simulink model "Channelizer_rb_v1"  (R2023b)
settings: Solver=VariableStepAuto  StartTime=0.0  StopTime=2048  RelTol=1e-3
PostLoadFcn:
  | TT = numerictype(1,16,15);
  | FF = fimath('RoundingMethod','Nearest','OverflowAction','Saturate');
  | mdl = channelizer_init(TT, FF);
  | channelizer = channelizer_model(mdl, TT, FF );
  | ch15 = 1; ch14 = ch15; ch13 = ch14; ch12 = ch13;
  | ch11 = ch12; ch10 = ch11; ch9 = ch10; ch8 = ch9;
  | ch7 = ch8; ch6 = ch7; ch5 = ch6; ch4 = ch5;
  | ch3 = ch4; ch2 = ch3; ch1 = ch2; ch0 = ch1;
undefined symbols (not defined in the file or in its folder): S, vsva2197, xcvc1902
libraries: aieUtilities x39, aieBasic x34, commrflib2 x16, commfilt2 x16, hlsBasic x3, vmcUtilities x1, commchan3 x1, commrandsrc3 x1, commdigbbndam3 x1
(part 2 of 2)

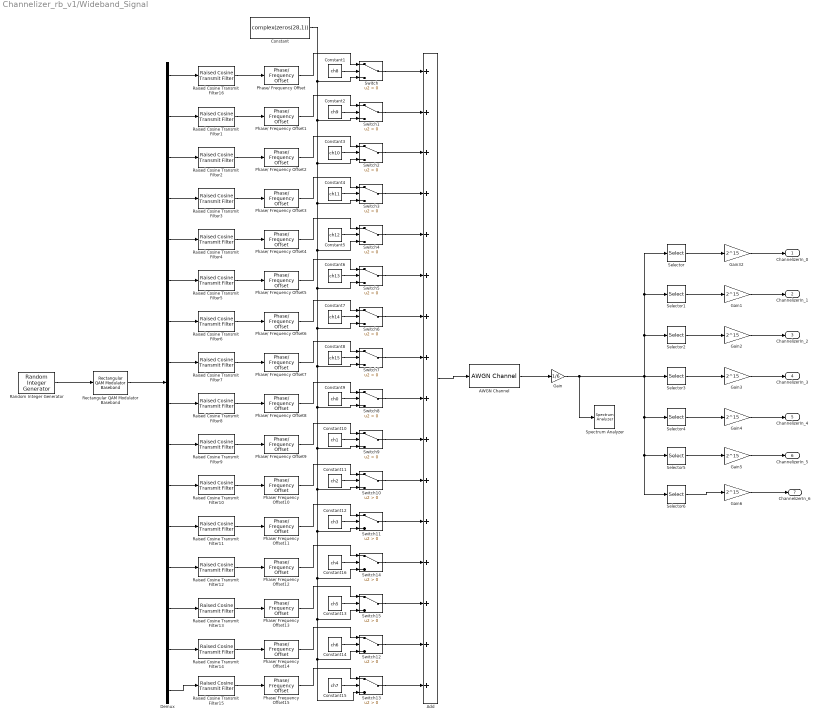
== system Channelizer_rb_v1/Wideband_Signal ==
  AWGN Channel : commchan3/AWGN Channel  LegacyMode=off  NoiseMethod="Signal to noise ratio  (SNR)"  noiseMode="Signal to noise ratio  (SNR)"  EbNo=10  EsNo=10  SNR=20  BitsPerSymbol=1  SignalPower=1  SamplesPerSymbol=1  SymbolPeriod=1  VarianceSource=Parameter  Variance=1  RandomStream=Global stream  Seed=67  SimulateUsing=Code generation
  Add : Sum  Inputs=++++++++++++++++
  Constant : Constant  Value=complex(zeros(28,1))
  Constant1 : Constant  Value=ch8
  Constant10 : Constant  Value=ch1
  Constant11 : Constant  Value=ch2
  Constant12 : Constant  Value=ch3
  Constant13 : Constant  Value=ch5
  Constant14 : Constant  Value=ch6
  Constant15 : Constant  Value=ch7
  Constant16 : Constant  Value=ch4
  Constant2 : Constant  Value=ch9
  Constant3 : Constant  Value=ch10
  Constant4 : Constant  Value=ch11
  Constant5 : Constant  Value=ch12
  Constant6 : Constant  Value=ch13
  Constant7 : Constant  Value=ch14
  Constant8 : Constant  Value=ch15
  Constant9 : Constant  Value=ch0
  Demux : Demux  Outputs=16
  Gain : Gain  Gain=1/6
  Gain{1..6,32} (7 alike) : Gain  Gain=2^15  OutDataTypeStr=int16
  Phase/ Frequency Offset : commrflib2/Phase// Frequency Offset  phaseOffset=0  freqPort=off  freqOffset=-8 * 8.75e9 / 16
  Phase/ Frequency Offset1 : commrflib2/Phase// Frequency Offset  phaseOffset=0  freqPort=off  freqOffset=-7 * 8.75e9 / 16
  Phase/ Frequency Offset10 : commrflib2/Phase// Frequency Offset  phaseOffset=0  freqPort=off  freqOffset=2 * 8.75e9 / 16
  Phase/ Frequency Offset11 : commrflib2/Phase// Frequency Offset  phaseOffset=0  freqPort=off  freqOffset=3 * 8.75e9 / 16
  Phase/ Frequency Offset12 : commrflib2/Phase// Frequency Offset  phaseOffset=0  freqPort=off  freqOffset=4 * 8.75e9 / 16
  Phase/ Frequency Offset13 : commrflib2/Phase// Frequency Offset  phaseOffset=0  freqPort=off  freqOffset=5 * 8.75e9 / 16
  Phase/ Frequency Offset14 : commrflib2/Phase// Frequency Offset  phaseOffset=0  freqPort=off  freqOffset=6 * 8.75e9 / 16
  Phase/ Frequency Offset15 : commrflib2/Phase// Frequency Offset  phaseOffset=0  freqPort=off  freqOffset=7 * 8.75e9 / 16
  Phase/ Frequency Offset2 : commrflib2/Phase// Frequency Offset  phaseOffset=0  freqPort=off  freqOffset=-6 * 8.75e9 / 16
  Phase/ Frequency Offset3 : commrflib2/Phase// Frequency Offset  phaseOffset=0  freqPort=off  freqOffset=-5 * 8.75e9 / 16
  Phase/ Frequency Offset4 : commrflib2/Phase// Frequency Offset  phaseOffset=0  freqPort=off  freqOffset=-4 * 8.75e9 / 16
  Phase/ Frequency Offset5 : commrflib2/Phase// Frequency Offset  phaseOffset=0  freqPort=off  freqOffset=-3 * 8.75e9 / 16
  Phase/ Frequency Offset6 : commrflib2/Phase// Frequency Offset  phaseOffset=0  freqPort=off  freqOffset=-2 * 8.75e9 / 16
  Phase/ Frequency Offset7 : commrflib2/Phase// Frequency Offset  phaseOffset=0  freqPort=off  freqOffset=-1 * 8.75e9 / 16
  Phase/ Frequency Offset8 : commrflib2/Phase// Frequency Offset  phaseOffset=0  freqPort=off  freqOffset=0 * 8.75e9 / 16
  Phase/ Frequency Offset9 : commrflib2/Phase// Frequency Offset  phaseOffset=0  freqPort=off  freqOffset=1 * 8.75e9 / 16
  Raised Cosine Transmit Filter1 : commfilt2/Raised Cosine Transmit Filter  filtType=Normal  R=0.3  filtSpan=10  N=28  filterGain=1  InputProcessing=Columns as channels (frame based)  RateOptions=Enforce single-rate processing  framing=Mute  checkCoeff=off  variableName=rcTxFilt1  checkGain=Normalized  sampMode=Mute  saveAsFlag=0  currentFiltSpan=10  D=(10)/2  launchFVT=on  roundingMode=Floor  overflowMode=off  coeffDataTypeStr=Inherit: Same word length as input  coeffMin=[]  coeffMax=[]  coeffLastDataTypeStr=Inherit: Same word length as input  outputDataTypeStr=Inherit: Same as accumulator  outputMin=[]  outputMax=[]  outputLastDataTypeStr=Inherit: Same as accumulator
  Raised Cosine Transmit Filter10 : commfilt2/Raised Cosine Transmit Filter  filtType=Normal  R=0.3  filtSpan=10  N=28  filterGain=1  InputProcessing=Columns as channels (frame based)  RateOptions=Enforce single-rate processing  framing=Mute  checkCoeff=off  variableName=rcTxFilt10  checkGain=Normalized  sampMode=Mute  saveAsFlag=0  currentFiltSpan=10  D=(10)/2  launchFVT=on  roundingMode=Floor  overflowMode=off  coeffDataTypeStr=Inherit: Same word length as input  coeffMin=[]  coeffMax=[]  coeffLastDataTypeStr=Inherit: Same word length as input  outputDataTypeStr=Inherit: Same as accumulator  outputMin=[]  outputMax=[]  outputLastDataTypeStr=Inherit: Same as accumulator
  Raised Cosine Transmit Filter11 : commfilt2/Raised Cosine Transmit Filter  filtType=Normal  R=0.3  filtSpan=10  N=28  filterGain=1  InputProcessing=Columns as channels (frame based)  RateOptions=Enforce single-rate processing  framing=Mute  checkCoeff=off  variableName=rcTxFilt11  checkGain=Normalized  sampMode=Mute  saveAsFlag=0  currentFiltSpan=10  D=(10)/2  launchFVT=on  roundingMode=Floor  overflowMode=off  coeffDataTypeStr=Inherit: Same word length as input  coeffMin=[]  coeffMax=[]  coeffLastDataTypeStr=Inherit: Same word length as input  outputDataTypeStr=Inherit: Same as accumulator  outputMin=[]  outputMax=[]  outputLastDataTypeStr=Inherit: Same as accumulator
  Raised Cosine Transmit Filter12 : commfilt2/Raised Cosine Transmit Filter  filtType=Normal  R=0.3  filtSpan=10  N=28  filterGain=1  InputProcessing=Columns as channels (frame based)  RateOptions=Enforce single-rate processing  framing=Mute  checkCoeff=off  variableName=rcTxFilt12  checkGain=Normalized  sampMode=Mute  saveAsFlag=0  currentFiltSpan=10  D=(10)/2  launchFVT=on  roundingMode=Floor  overflowMode=off  coeffDataTypeStr=Inherit: Same word length as input  coeffMin=[]  coeffMax=[]  coeffLastDataTypeStr=Inherit: Same word length as input  outputDataTypeStr=Inherit: Same as accumulator  outputMin=[]  outputMax=[]  outputLastDataTypeStr=Inherit: Same as accumulator
  Raised Cosine Transmit Filter13 : commfilt2/Raised Cosine Transmit Filter  filtType=Normal  R=0.3  filtSpan=10  N=28  filterGain=1  InputProcessing=Columns as channels (frame based)  RateOptions=Enforce single-rate processing  framing=Mute  checkCoeff=off  variableName=rcTxFilt13  checkGain=Normalized  sampMode=Mute  saveAsFlag=0  currentFiltSpan=10  D=(10)/2  launchFVT=on  roundingMode=Floor  overflowMode=off  coeffDataTypeStr=Inherit: Same word length as input  coeffMin=[]  coeffMax=[]  coeffLastDataTypeStr=Inherit: Same word length as input  outputDataTypeStr=Inherit: Same as accumulator  outputMin=[]  outputMax=[]  outputLastDataTypeStr=Inherit: Same as accumulator
  Raised Cosine Transmit Filter14 : commfilt2/Raised Cosine Transmit Filter  filtType=Normal  R=0.3  filtSpan=10  N=28  filterGain=1  InputProcessing=Columns as channels (frame based)  RateOptions=Enforce single-rate processing  framing=Mute  checkCoeff=off  variableName=rcTxFilt14  checkGain=Normalized  sampMode=Mute  saveAsFlag=0  currentFiltSpan=10  D=(10)/2  launchFVT=on  roundingMode=Floor  overflowMode=off  coeffDataTypeStr=Inherit: Same word length as input  coeffMin=[]  coeffMax=[]  coeffLastDataTypeStr=Inherit: Same word length as input  outputDataTypeStr=Inherit: Same as accumulator  outputMin=[]  outputMax=[]  outputLastDataTypeStr=Inherit: Same as accumulator
  Raised Cosine Transmit Filter15 : commfilt2/Raised Cosine Transmit Filter  filtType=Normal  R=0.3  filtSpan=10  N=28  filterGain=1  InputProcessing=Columns as channels (frame based)  RateOptions=Enforce single-rate processing  framing=Mute  checkCoeff=off  variableName=rcTxFilt15  checkGain=Normalized  sampMode=Mute  saveAsFlag=0  currentFiltSpan=10  D=(10)/2  launchFVT=on  roundingMode=Floor  overflowMode=off  coeffDataTypeStr=Inherit: Same word length as input  coeffMin=[]  coeffMax=[]  coeffLastDataTypeStr=Inherit: Same word length as input  outputDataTypeStr=Inherit: Same as accumulator  outputMin=[]  outputMax=[]  outputLastDataTypeStr=Inherit: Same as accumulator
  Raised Cosine Transmit Filter16 : commfilt2/Raised Cosine Transmit Filter  filtType=Normal  R=0.3  filtSpan=10  N=28  filterGain=1  InputProcessing=Columns as channels (frame based)  RateOptions=Enforce single-rate processing  framing=Mute  checkCoeff=off  variableName=rcTxFilt16  checkGain=Normalized  sampMode=Mute  saveAsFlag=0  currentFiltSpan=10  D=(10)/2  launchFVT=on  roundingMode=Floor  overflowMode=off  coeffDataTypeStr=Inherit: Same word length as input  coeffMin=[]  coeffMax=[]  coeffLastDataTypeStr=Inherit: Same word length as input  outputDataTypeStr=Inherit: Same as accumulator  outputMin=[]  outputMax=[]  outputLastDataTypeStr=Inherit: Same as accumulator
  Raised Cosine Transmit Filter2 : commfilt2/Raised Cosine Transmit Filter  filtType=Normal  R=0.3  filtSpan=10  N=28  filterGain=1  InputProcessing=Columns as channels (frame based)  RateOptions=Enforce single-rate processing  framing=Mute  checkCoeff=off  variableName=rcTxFilt2  checkGain=Normalized  sampMode=Mute  saveAsFlag=0  currentFiltSpan=10  D=(10)/2  launchFVT=on  roundingMode=Floor  overflowMode=off  coeffDataTypeStr=Inherit: Same word length as input  coeffMin=[]  coeffMax=[]  coeffLastDataTypeStr=Inherit: Same word length as input  outputDataTypeStr=Inherit: Same as accumulator  outputMin=[]  outputMax=[]  outputLastDataTypeStr=Inherit: Same as accumulator
  Raised Cosine Transmit Filter3 : commfilt2/Raised Cosine Transmit Filter  filtType=Normal  R=0.3  filtSpan=10  N=28  filterGain=1  InputProcessing=Columns as channels (frame based)  RateOptions=Enforce single-rate processing  framing=Mute  checkCoeff=off  variableName=rcTxFilt3  checkGain=Normalized  sampMode=Mute  saveAsFlag=0  currentFiltSpan=10  D=(10)/2  launchFVT=on  roundingMode=Floor  overflowMode=off  coeffDataTypeStr=Inherit: Same word length as input  coeffMin=[]  coeffMax=[]  coeffLastDataTypeStr=Inherit: Same word length as input  outputDataTypeStr=Inherit: Same as accumulator  outputMin=[]  outputMax=[]  outputLastDataTypeStr=Inherit: Same as accumulator
  Raised Cosine Transmit Filter4 : commfilt2/Raised Cosine Transmit Filter  filtType=Normal  R=0.3  filtSpan=10  N=28  filterGain=1  InputProcessing=Columns as channels (frame based)  RateOptions=Enforce single-rate processing  framing=Mute  checkCoeff=off  variableName=rcTxFilt4  checkGain=Normalized  sampMode=Mute  saveAsFlag=0  currentFiltSpan=10  D=(10)/2  launchFVT=on  roundingMode=Floor  overflowMode=off  coeffDataTypeStr=Inherit: Same word length as input  coeffMin=[]  coeffMax=[]  coeffLastDataTypeStr=Inherit: Same word length as input  outputDataTypeStr=Inherit: Same as accumulator  outputMin=[]  outputMax=[]  outputLastDataTypeStr=Inherit: Same as accumulator
  Raised Cosine Transmit Filter5 : commfilt2/Raised Cosine Transmit Filter  filtType=Normal  R=0.3  filtSpan=10  N=28  filterGain=1  InputProcessing=Columns as channels (frame based)  RateOptions=Enforce single-rate processing  framing=Mute  checkCoeff=off  variableName=rcTxFilt5  checkGain=Normalized  sampMode=Mute  saveAsFlag=0  currentFiltSpan=10  D=(10)/2  launchFVT=on  roundingMode=Floor  overflowMode=off  coeffDataTypeStr=Inherit: Same word length as input  coeffMin=[]  coeffMax=[]  coeffLastDataTypeStr=Inherit: Same word length as input  outputDataTypeStr=Inherit: Same as accumulator  outputMin=[]  outputMax=[]  outputLastDataTypeStr=Inherit: Same as accumulator
  Raised Cosine Transmit Filter6 : commfilt2/Raised Cosine Transmit Filter  filtType=Normal  R=0.3  filtSpan=10  N=28  filterGain=1  InputProcessing=Columns as channels (frame based)  RateOptions=Enforce single-rate processing  framing=Mute  checkCoeff=off  variableName=rcTxFilt6  checkGain=Normalized  sampMode=Mute  saveAsFlag=0  currentFiltSpan=10  D=(10)/2  launchFVT=on  roundingMode=Floor  overflowMode=off  coeffDataTypeStr=Inherit: Same word length as input  coeffMin=[]  coeffMax=[]  coeffLastDataTypeStr=Inherit: Same word length as input  outputDataTypeStr=Inherit: Same as accumulator  outputMin=[]  outputMax=[]  outputLastDataTypeStr=Inherit: Same as accumulator
  Raised Cosine Transmit Filter7 : commfilt2/Raised Cosine Transmit Filter  filtType=Normal  R=0.3  filtSpan=10  N=28  filterGain=1  InputProcessing=Columns as channels (frame based)  RateOptions=Enforce single-rate processing  framing=Mute  checkCoeff=off  variableName=rcTxFilt7  checkGain=Normalized  sampMode=Mute  saveAsFlag=0  currentFiltSpan=10  D=(10)/2  launchFVT=on  roundingMode=Floor  overflowMode=off  coeffDataTypeStr=Inherit: Same word length as input  coeffMin=[]  coeffMax=[]  coeffLastDataTypeStr=Inherit: Same word length as input  outputDataTypeStr=Inherit: Same as accumulator  outputMin=[]  outputMax=[]  outputLastDataTypeStr=Inherit: Same as accumulator
  Raised Cosine Transmit Filter8 : commfilt2/Raised Cosine Transmit Filter  filtType=Normal  R=0.3  filtSpan=10  N=28  filterGain=1  InputProcessing=Columns as channels (frame based)  RateOptions=Enforce single-rate processing  framing=Mute  checkCoeff=off  variableName=rcTxFilt8  checkGain=Normalized  sampMode=Mute  saveAsFlag=0  currentFiltSpan=10  D=(10)/2  launchFVT=on  roundingMode=Floor  overflowMode=off  coeffDataTypeStr=Inherit: Same word length as input  coeffMin=[]  coeffMax=[]  coeffLastDataTypeStr=Inherit: Same word length as input  outputDataTypeStr=Inherit: Same as accumulator  outputMin=[]  outputMax=[]  outputLastDataTypeStr=Inherit: Same as accumulator
  Raised Cosine Transmit Filter9 : commfilt2/Raised Cosine Transmit Filter  filtType=Normal  R=0.3  filtSpan=10  N=28  filterGain=1  InputProcessing=Columns as channels (frame based)  RateOptions=Enforce single-rate processing  framing=Mute  checkCoeff=off  variableName=rcTxFilt9  checkGain=Normalized  sampMode=Mute  saveAsFlag=0  currentFiltSpan=10  D=(10)/2  launchFVT=on  roundingMode=Floor  overflowMode=off  coeffDataTypeStr=Inherit: Same word length as input  coeffMin=[]  coeffMax=[]  coeffLastDataTypeStr=Inherit: Same word length as input  outputDataTypeStr=Inherit: Same as accumulator  outputMin=[]  outputMax=[]  outputLastDataTypeStr=Inherit: Same as accumulator
  Random Integer Generator : commrandsrc3/Random Integer Generator  SetSize=16  SeedSource=Auto  Seed=0  SampleTime=(7/4)/8.75e9  SamplesPerFrame=16  OutputDataType=double  SimulateUsing=Interpreted execution
  Rectangular QAM Modulator Baseband : commdigbbndam3/Rectangular QAM Modulator Baseband  M=16  InType=Integer  Enc=Gray  Mapping=[0:15]  PowType=Min. distance between symbols  MinDist=2  AvgPow=1  PeakPow=1  Ph=0  outDtype=double  outWordLen=16  outUDDataType=sfix(16)  outFracLenMode=Best precision  outFracLen=15  outDataTypeStr=double  outLastDataTypeStr=double
  Selector : Selector  InputPortWidth=28  IndexOptions=Index vector (dialog)  Indices=[14 7 28 21]  OutputSizes=1
  Selector1 : Selector  InputPortWidth=28  IndexOptions=Index vector (dialog)  Indices=[13 6 27 20]  OutputSizes=1
  Selector2 : Selector  InputPortWidth=28  IndexOptions=Index vector (dialog)  Indices=[12 5 26 19]  OutputSizes=1
  Selector3 : Selector  InputPortWidth=28  IndexOptions=Index vector (dialog)  Indices=[11 4 25 18]  OutputSizes=1
  Selector4 : Selector  InputPortWidth=28  IndexOptions=Index vector (dialog)  Indices=[10 3 24 17]  OutputSizes=1
  Selector5 : Selector  InputPortWidth=28  IndexOptions=Index vector (dialog)  Indices=[9 2 23 16]  OutputSizes=1
  Selector6 : Selector  InputPortWidth=28  IndexOptions=Index vector (dialog)  Indices=[8 1 22 15]  OutputSizes=1
  Spectrum Analyzer : SpectrumAnalyzer  WindowPosition=[372.000000,752.000000,800.000000,500.000000,]  Visible=on  ScopeFrameLocation=window  SpectrumType=Power density  ViewType=Spectrum and spectrogram  Span=8750000000  StartFrequency=-4375000000  StopFrequency=4375000000  AveragingMethod=Exponential  SpectrumUnits=dBm/Hz  YLimits=[-113.07087449,-68.64016986]  ColorLimits=[-113.07087449,-68.64016986]
  Switch{,1..15} (16 alike) : Switch  Criteria=u2 > Threshold  SaturateOnIntegerOverflow=off  InputSameDT=off
  ChannelizerIn_0 : Outport
  ChannelizerIn_1 : Outport  Port=2
  ChannelizerIn_2 : Outport  Port=3
  ChannelizerIn_3 : Outport  Port=4
  ChannelizerIn_4 : Outport  Port=5
  ChannelizerIn_5 : Outport  Port=6
  ChannelizerIn_6 : Outport  Port=7
  wires:
  Random Integer Generator/1 -> Rectangular QAM Modulator Baseband/1
  Rectangular QAM Modulator Baseband/1 -> Demux/1
  Demux/1 -> Raised Cosine Transmit Filter16/1
  Demux/2 -> Raised Cosine Transmit Filter1/1
  Demux/4 -> Raised Cosine Transmit Filter3/1
  Demux/3 -> Raised Cosine Transmit Filter2/1
  Demux/5 -> Raised Cosine Transmit Filter4/1
  Demux/6 -> Raised Cosine Transmit Filter5/1
  Demux/7 -> Raised Cosine Transmit Filter6/1
  Demux/8 -> Raised Cosine Transmit Filter7/1
  Demux/16 -> Raised Cosine Transmit Filter15/1
  Demux/15 -> Raised Cosine Transmit Filter14/1
  Demux/14 -> Raised Cosine Transmit Filter13/1
  Demux/13 -> Raised Cosine Transmit Filter12/1
  Demux/12 -> Raised Cosine Transmit Filter11/1
  Demux/11 -> Raised Cosine Transmit Filter10/1
  Demux/10 -> Raised Cosine Transmit Filter9/1
  Demux/9 -> Raised Cosine Transmit Filter8/1
  Raised Cosine Transmit Filter16/1 -> Phase/ Frequency Offset/1
  Raised Cosine Transmit Filter1/1 -> Phase/ Frequency Offset1/1
  Raised Cosine Transmit Filter2/1 -> Phase/ Frequency Offset2/1
  Raised Cosine Transmit Filter3/1 -> Phase/ Frequency Offset3/1
  Raised Cosine Transmit Filter4/1 -> Phase/ Frequency Offset4/1
  Raised Cosine Transmit Filter5/1 -> Phase/ Frequency Offset5/1
  Raised Cosine Transmit Filter6/1 -> Phase/ Frequency Offset6/1
  Raised Cosine Transmit Filter7/1 -> Phase/ Frequency Offset7/1
  Raised Cosine Transmit Filter8/1 -> Phase/ Frequency Offset8/1
  Raised Cosine Transmit Filter9/1 -> Phase/ Frequency Offset9/1
  Raised Cosine Transmit Filter10/1 -> Phase/ Frequency Offset10/1
  Raised Cosine Transmit Filter11/1 -> Phase/ Frequency Offset11/1
  Raised Cosine Transmit Filter12/1 -> Phase/ Frequency Offset12/1
  Raised Cosine Transmit Filter13/1 -> Phase/ Frequency Offset13/1
  Raised Cosine Transmit Filter14/1 -> Phase/ Frequency Offset14/1
  Raised Cosine Transmit Filter15/1 -> Phase/ Frequency Offset15/1
  Add/1 -> AWGN Channel/1
  AWGN Channel/1 -> Gain/1
  Switch/1 -> Add/1
  Constant1/1 -> Switch/2
  Constant2/1 -> Switch1/2
  Switch1/1 -> Add/2
  Constant3/1 -> Switch2/2
  Switch2/1 -> Add/3
  Constant4/1 -> Switch3/2
  Switch3/1 -> Add/4
  Switch5/1 -> Add/6
  Constant6/1 -> Switch5/2
  Switch6/1 -> Add/7
  Constant7/1 -> Switch6/2
  Switch7/1 -> Add/8
  Switch4/1 -> Add/5
  Constant8/1 -> Switch7/2
  Constant5/1 -> Switch4/2
  Constant10/1 -> Switch9/2
  Switch11/1 -> Add/12
  Switch9/1 -> Add/10
  Constant11/1 -> Switch10/2
  Constant12/1 -> Switch11/2
  Constant9/1 -> Switch8/2
  Switch10/1 -> Add/11
  Switch8/1 -> Add/9
  Constant15/1 -> Switch13/2
  Switch12/1 -> Add/15
  Switch13/1 -> Add/16
  Switch14/1 -> Add/13
  Switch15/1 -> Add/14
  Constant16/1 -> Switch14/2
  Constant14/1 -> Switch12/2
  Constant13/1 -> Switch15/2
  Phase/ Frequency Offset15/1 -> Switch13/1
  Phase/ Frequency Offset14/1 -> Switch12/1
  Phase/ Frequency Offset13/1 -> Switch15/1
  Phase/ Frequency Offset12/1 -> Switch14/1
  Phase/ Frequency Offset11/1 -> Switch11/1
  Phase/ Frequency Offset10/1 -> Switch10/1
  Phase/ Frequency Offset9/1 -> Switch9/1
  Phase/ Frequency Offset8/1 -> Switch8/1
  Phase/ Frequency Offset7/1 -> Switch7/1
  Phase/ Frequency Offset6/1 -> Switch6/1
  Phase/ Frequency Offset5/1 -> Switch5/1
  Phase/ Frequency Offset4/1 -> Switch4/1
  Phase/ Frequency Offset3/1 -> Switch3/1
  Phase/ Frequency Offset2/1 -> Switch2/1
  Phase/ Frequency Offset1/1 -> Switch1/1
  Phase/ Frequency Offset/1 -> Switch/1
  Constant/1 -> Switch/3, Switch1/3, Switch2/3, Switch3/3, Switch4/3, Switch5/3, Switch6/3, Switch7/3, Switch8/3, Switch9/3, Switch10/3, Switch11/3, Switch14/3, Switch15/3, Switch12/3, Switch13/3
  Gain/1 -> Selector3/1, Selector4/1, Selector5/1, Selector6/1, Selector2/1, Selector1/1, Selector/1, Spectrum Analyzer/1
  Selector/1 -> Gain32/1
  Gain32/1 -> ChannelizerIn_0/1
  Selector1/1 -> Gain1/1
  Selector2/1 -> Gain2/1
  Selector4/1 -> Gain4/1
  Selector3/1 -> Gain3/1
  Selector6/1 -> Gain6/1
  Selector5/1 -> Gain5/1
  Gain1/1 -> ChannelizerIn_1/1
  Gain2/1 -> ChannelizerIn_2/1
  Gain3/1 -> ChannelizerIn_3/1
  Gain4/1 -> ChannelizerIn_4/1
  Gain5/1 -> ChannelizerIn_5/1
  Gain6/1 -> ChannelizerIn_6/1

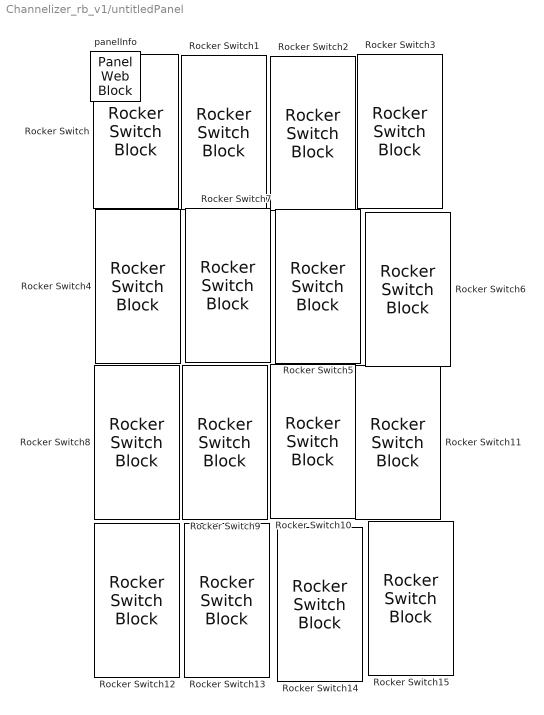
== system Channelizer_rb_v1/untitledPanel ==
  Rocker Switch : RockerSwitchBlock  Tag=HiddenForWebPanel  PanelInfo="{\"addnFilesFolder\":\"\",\"height\":154,\"includeDebugPackages\":false,\"left\":10,\"outputFolder\":\"\",\"panelId\":\"panelId-fec1c322-f5e7-4e4f-8c31-b98d6132c1cd\",\"popoutMode\":\"\",\"standaloneTitle\":\"\",\"top\":12,\"type\":\"panelChild\",\"version\":\"2019b\",\"width\":85,\"zIndex\":1500002}"
      settings: Values={{'Off', 'On'}, [0 1]}
  Rocker Switch1 : RockerSwitchBlock  Tag=HiddenForWebPanel  PanelInfo="{\"addnFilesFolder\":\"\",\"height\":154,\"includeDebugPackages\":false,\"left\":98,\"outputFolder\":\"\",\"panelId\":\"panelId-fec1c322-f5e7-4e4f-8c31-b98d6132c1cd\",\"popoutMode\":\"\",\"standaloneTitle\":\"\",\"top\":12,\"type\":\"panelChild\",\"version\":\"2019b\",\"width\":85,\"zIndex\":1500004}"
      settings: Values={{'Off', 'On'}, [0 1]}
  Rocker Switch10 : RockerSwitchBlock  Tag=HiddenForWebPanel  PanelInfo="{\"addnFilesFolder\":\"\",\"height\":154,\"includeDebugPackages\":false,\"left\":185,\"outputFolder\":\"\",\"panelId\":\"panelId-fec1c322-f5e7-4e4f-8c31-b98d6132c1cd\",\"popoutMode\":\"\",\"standaloneTitle\":\"\",\"top\":327,\"type\":\"panelChild\",\"version\":\"2019b\",\"width\":85,\"zIndex\":1500022}"
      settings: Values={{'Off', 'On'}, [0 1]}
  Rocker Switch11 : RockerSwitchBlock  Tag=HiddenForWebPanel  PanelInfo="{\"addnFilesFolder\":\"\",\"height\":154,\"includeDebugPackages\":false,\"left\":273,\"outputFolder\":\"\",\"panelId\":\"panelId-fec1c322-f5e7-4e4f-8c31-b98d6132c1cd\",\"popoutMode\":\"\",\"standaloneTitle\":\"\",\"top\":327,\"type\":\"panelChild\",\"version\":\"2019b\",\"width\":85,\"zIndex\":1500024}"
      settings: Values={{'Off', 'On'}, [0 1]}
  Rocker Switch12 : RockerSwitchBlock  Tag=HiddenForWebPanel  PanelInfo="{\"addnFilesFolder\":\"\",\"height\":154,\"includeDebugPackages\":false,\"left\":10,\"outputFolder\":\"\",\"panelId\":\"panelId-fec1c322-f5e7-4e4f-8c31-b98d6132c1cd\",\"popoutMode\":\"\",\"standaloneTitle\":\"\",\"top\":483,\"type\":\"panelChild\",\"version\":\"2019b\",\"width\":85,\"zIndex\":1500026}"
      settings: Values={{'Off', 'On'}, [0 1]}
  Rocker Switch13 : RockerSwitchBlock  Tag=HiddenForWebPanel  PanelInfo="{\"addnFilesFolder\":\"\",\"height\":154,\"includeDebugPackages\":false,\"left\":97,\"outputFolder\":\"\",\"panelId\":\"panelId-fec1c322-f5e7-4e4f-8c31-b98d6132c1cd\",\"popoutMode\":\"\",\"standaloneTitle\":\"\",\"top\":483,\"type\":\"panelChild\",\"version\":\"2019b\",\"width\":85,\"zIndex\":1500028}"
      settings: Values={{'Off', 'On'}, [0 1]}
  Rocker Switch14 : RockerSwitchBlock  Tag=HiddenForWebPanel  PanelInfo="{\"addnFilesFolder\":\"\",\"height\":154,\"includeDebugPackages\":false,\"left\":185,\"outputFolder\":\"\",\"panelId\":\"panelId-fec1c322-f5e7-4e4f-8c31-b98d6132c1cd\",\"popoutMode\":\"\",\"standaloneTitle\":\"\",\"top\":484,\"type\":\"panelChild\",\"version\":\"2019b\",\"width\":85,\"zIndex\":1500030}"
      settings: Values={{'Off', 'On'}, [0 1]}
  Rocker Switch15 : RockerSwitchBlock  Tag=HiddenForWebPanel  PanelInfo="{\"addnFilesFolder\":\"\",\"height\":154,\"includeDebugPackages\":false,\"left\":272,\"outputFolder\":\"\",\"panelId\":\"panelId-fec1c322-f5e7-4e4f-8c31-b98d6132c1cd\",\"popoutMode\":\"\",\"standaloneTitle\":\"\",\"top\":484,\"type\":\"panelChild\",\"version\":\"2019b\",\"width\":85,\"zIndex\":1500032}"
      settings: Values={{'Off', 'On'}, [0 1]}
  Rocker Switch2 : RockerSwitchBlock  Tag=HiddenForWebPanel  PanelInfo="{\"addnFilesFolder\":\"\",\"height\":154,\"includeDebugPackages\":false,\"left\":186,\"outputFolder\":\"\",\"panelId\":\"panelId-fec1c322-f5e7-4e4f-8c31-b98d6132c1cd\",\"popoutMode\":\"\",\"standaloneTitle\":\"\",\"top\":12,\"type\":\"panelChild\",\"version\":\"2019b\",\"width\":85,\"zIndex\":1500006}"
      settings: Values={{'Off', 'On'}, [0 1]}
  Rocker Switch3 : RockerSwitchBlock  Tag=HiddenForWebPanel  PanelInfo="{\"addnFilesFolder\":\"\",\"height\":154,\"includeDebugPackages\":false,\"left\":274,\"outputFolder\":\"\",\"panelId\":\"panelId-fec1c322-f5e7-4e4f-8c31-b98d6132c1cd\",\"popoutMode\":\"\",\"standaloneTitle\":\"\",\"top\":12,\"type\":\"panelChild\",\"version\":\"2019b\",\"width\":85,\"zIndex\":1500008}"
      settings: Values={{'Off', 'On'}, [0 1]}
  Rocker Switch4 : RockerSwitchBlock  Tag=HiddenForWebPanel  PanelInfo="{\"addnFilesFolder\":\"\",\"height\":154,\"includeDebugPackages\":false,\"left\":10,\"outputFolder\":\"\",\"panelId\":\"panelId-fec1c322-f5e7-4e4f-8c31-b98d6132c1cd\",\"popoutMode\":\"\",\"standaloneTitle\":\"\",\"top\":169,\"type\":\"panelChild\",\"version\":\"2019b\",\"width\":85,\"zIndex\":1500010}"
      settings: Values={{'Off', 'On'}, [0 1]}
  Rocker Switch5 : RockerSwitchBlock  Tag=HiddenForWebPanel  PanelInfo="{\"addnFilesFolder\":\"\",\"height\":154,\"includeDebugPackages\":false,\"left\":186,\"outputFolder\":\"\",\"panelId\":\"panelId-fec1c322-f5e7-4e4f-8c31-b98d6132c1cd\",\"popoutMode\":\"\",\"standaloneTitle\":\"\",\"top\":170,\"type\":\"panelChild\",\"version\":\"2019b\",\"width\":85,\"zIndex\":1500012}"
      settings: Values={{'Off', 'On'}, [0 1]}
  Rocker Switch6 : RockerSwitchBlock  Tag=HiddenForWebPanel  PanelInfo="{\"addnFilesFolder\":\"\",\"height\":154,\"includeDebugPackages\":false,\"left\":274,\"outputFolder\":\"\",\"panelId\":\"panelId-fec1c322-f5e7-4e4f-8c31-b98d6132c1cd\",\"popoutMode\":\"\",\"standaloneTitle\":\"\",\"top\":170,\"type\":\"panelChild\",\"version\":\"2019b\",\"width\":85,\"zIndex\":1500014}"
      settings: Values={{'Off', 'On'}, [0 1]}
  Rocker Switch7 : RockerSwitchBlock  Tag=HiddenForWebPanel  PanelInfo="{\"addnFilesFolder\":\"\",\"height\":154,\"includeDebugPackages\":false,\"left\":98,\"outputFolder\":\"\",\"panelId\":\"panelId-fec1c322-f5e7-4e4f-8c31-b98d6132c1cd\",\"popoutMode\":\"\",\"standaloneTitle\":\"\",\"top\":169,\"type\":\"panelChild\",\"version\":\"2019b\",\"width\":85,\"zIndex\":1500016}"
      settings: Values={{'Off', 'On'}, [0 1]}
  Rocker Switch8 : RockerSwitchBlock  Tag=HiddenForWebPanel  PanelInfo="{\"addnFilesFolder\":\"\",\"height\":154,\"includeDebugPackages\":false,\"left\":10,\"outputFolder\":\"\",\"panelId\":\"panelId-fec1c322-f5e7-4e4f-8c31-b98d6132c1cd\",\"popoutMode\":\"\",\"standaloneTitle\":\"\",\"top\":326,\"type\":\"panelChild\",\"version\":\"2019b\",\"width\":85,\"zIndex\":1500018}"
      settings: Values={{'Off', 'On'}, [0 1]}
  Rocker Switch9 : RockerSwitchBlock  Tag=HiddenForWebPanel  PanelInfo="{\"addnFilesFolder\":\"\",\"height\":154,\"includeDebugPackages\":false,\"left\":97,\"outputFolder\":\"\",\"panelId\":\"panelId-fec1c322-f5e7-4e4f-8c31-b98d6132c1cd\",\"popoutMode\":\"\",\"standaloneTitle\":\"\",\"top\":326,\"type\":\"panelChild\",\"version\":\"2019b\",\"width\":85,\"zIndex\":1500020}"
      settings: Values={{'Off', 'On'}, [0 1]}
  panelInfo : PanelWebBlock  Tag=HiddenForWebPanel  PanelInfo="{\"addnFilesFolder\":\"\",\"compacted\":false,\"height\":655,\"includeDebugPackages\":false,\"isActiveTab\":true,\"left\":82,\"name\":\"Panel\",\"outputFolder\":\"\",\"panelId\":\"panelId-fec1c322-f5e7-4e4f-8c31-b98d6132c1cd\",\"popoutMode\":\"\",\"standaloneTitle\":\"\",\"tabIndex\":0,\"tabbedSetId\":\"tabbedSet6868322055\",\"top\":471,\"type\":\"panel\",\"version\":\"2019b\",\"visible\":true,\"width\":371,\"zIndex\":1500002}"  PanelSnapshot=<binary blob, 10492 chars, not shown>

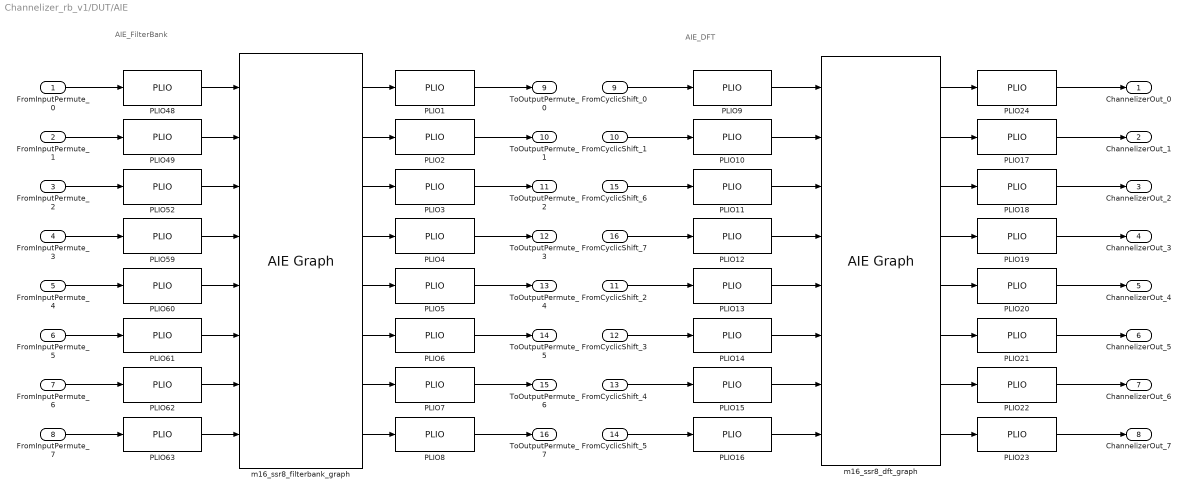
== system Channelizer_rb_v1/DUT/AIE ==
  note: AIE_DFT
  note: AIE_FilterBank
  FromInputPermute_0 : Inport
  FromInputPermute_1 : Inport  Port=2
  FromInputPermute_2 : Inport  Port=3
  FromInputPermute_3 : Inport  Port=4
  FromInputPermute_4 : Inport  Port=5
  FromInputPermute_5 : Inport  Port=6
  FromInputPermute_6 : Inport  Port=7
  FromInputPermute_7 : Inport  Port=8
  FromCyclicShift_0 : Inport  Port=9
  FromCyclicShift_1 : Inport  Port=10
  FromCyclicShift_2 : Inport  Port=11
  FromCyclicShift_3 : Inport  Port=12
  FromCyclicShift_4 : Inport  Port=13
  FromCyclicShift_5 : Inport  Port=14
  FromCyclicShift_6 : Inport  Port=15
  FromCyclicShift_7 : Inport  Port=16
  PLIO{1..24,48..49,52,59..63} (32 alike) : aieBasic/PLIO  PlioWidth=64  PlioFreqSpec=on  PlioFreq=625  ColLocation=0  channel=0  blockJsonConstraints=[]  deprecateConstraints=0
  m16_ssr8_dft_graph : aieBasic/AIE Graph  PortAttributesTable={ 'Input', 'sig_i[0]', 'stream', 'cint16', '', '', ''; 'Input', 'sig_i[1]', 'stream', 'cint16', '', '', ''; 'Input', 'sig_i[6]', 'stream', 'cint16', '', '', ''; 'Input', 'sig_i[7]', 'stream', 'cint16', '', '', ''; 'Input', 'sig_i[2]', 'stream', 'cint16', '', '', ''; 'Input', 'sig_i[3]', 'stream', 'cint16', '', '', ''; 'Input', 'sig_i[4]', 'stream', 'cint16', '', '', ''; 'Input', 'sig_i[5]', 'stream', 'cint16', '', '', ''; 'Output', 'sig_o[0]', 'stream', 'cint16', '', '', '4'; 'Output', 'sig_o[1]', 'stream', 'cint16', '', '', '4'; 'Output', 'sig_o[2]', 'stream', 'cint16', '', '', '4'; 'Output', 'sig_o[3]', 'stream', 'cint16', '', '', '4'; 'Output', 'sig_o[4]', 'stream', 'cint16', '', '', '4'; 'Output', 'sig_o[5]', 'stream', 'cint16', '', '', '4'; 'Output', 'sig_o[6]', 'stream', 'cint16', '', '', '4'; 'Output', 'sig_o[7]', 'stream', 'cint16', '', '', '4' }  PortAttributesEnablement={'off', 'on', 'off', 'off', 'off', 'off', 'off';'off', 'on', 'off', 'off', 'off', 'off', 'off';'off', 'on', 'off', 'off', 'off', 'off', 'off';'off', 'on', 'off', 'off', 'off', 'off', 'off';'off', 'on', 'off', 'off', 'off', 'off', 'off';'off', 'on', 'off', 'off', 'off', 'off', 'off';'off', 'on', 'off', 'off', 'off', 'off', 'off';'off', 'on', 'off', 'off', 'off', 'off', 'off';'off', 'on', 'off', 'off', 'off', 'off', 'on';'off', 'on', 'off', 'off', 'off', 'off', 'on';'off', 'on', 'off', 'off', 'off', 'off', 'on';'off', 'on', 'off', 'off', 'off', 'off', 'on';'off', 'on', 'off', 'off', 'off', 'off', 'on';'off', 'on', 'off', 'off', 'off', 'off', 'on';'off', 'on', 'off', 'off', 'off', 'off', 'on';'off', 'on', 'off', 'off', 'off', 'off', 'on'}  SampleTime=-1  ClassDeclTypeOptions=C[1 1]@t24@class m16_ssr8_dft_graph  ClassDecl=class m16_ssr8_dft_graph  ClassTemplateParams={}  ClassTemplateParamsEnables={}  ClassCtorDeclTypeOptions=C[1 1]@t7@<empty>  ClassCtorDecl=<empty>  ClassCtorParams={}  GraphAllAttrs=|  PortArgDecls={'in stream cint16 in1'; 'in stream cint16 in2'; 'in stream cint16 in3'; 'in stream cint16 in4'; 'in stream cint16 in5'; 'in stream cint16 in6'; 'in stream cint16 in7'; 'in stream cint16 in8'; 'out stream cint16 out1'; 'out stream cint16 out2'; 'out stream cint16 out3'; 'out stream cint16 out4'; 'out stream cint16 out5'; 'out stream cint16 out6'; 'out stream cint16 out7'; 'out stream cint16 out8'}  PortGraphPortNames={'sig_i[0]'; 'sig_i[1]'; 'sig_i[6]'; 'sig_i[7]'; 'sig_i[2]'; 'sig_i[3]'; 'sig_i[4]'; 'sig_i[5]'; 'sig_o[0]'; 'sig_o[1]'; 'sig_o[2]'; 'sig_o[3]'; 'sig_o[4]'; 'sig_o[5]'; 'sig_o[6]'; 'sig_o[7]'}  PortTypes={'stream'; 'stream'; 'stream'; 'stream'; 'stream'; 'stream'; 'stream'; 'stream'; 'stream'; 'stream'; 'stream'; 'stream'; 'stream'; 'stream'; 'stream'; 'stream'}  PortDataTypes={'cint16'; 'cint16'; 'cint16'; 'cint16'; 'cint16'; 'cint16'; 'cint16'; 'cint16'; 'cint16'; 'cint16'; 'cint16'; 'cint16'; 'cint16'; 'cint16'; 'cint16'; 'cint16'}  PortSizes={0.000000000000000000e+00; 0.000000000000000000e+00; 0.000000000000000000e+00; 0.000000000000000000e+00; 0.000000000000000000e+00; 0.000000000000000000e+00; 0.000000000000000000e+00; 0.000000000000000000e+00; 0.000000000000000000e+00; 0.000000000000000000e+00; 0.000000000000000000e+00; 0.000000000000000000e+00; 0.000000000000000000e+00; 0.000000000000000000e+00; 0.000000000000000000e+00; 0.000000000000000000e+00}  PortSynchronicities={'auto'; 'auto'; 'auto'; 'auto'; 'auto'; 'auto'; 'auto'; 'auto'; 'auto'; 'auto'; 'auto'; 'auto'; 'auto'; 'auto'; 'auto'; 'auto'}  PortSignalSizes={0.000000000000000000e+00; 0.000000000000000000e+00; 0.000000000000000000e+00; 0.000000000000000000e+00; 0.000000000000000000e+00; 0.000000000000000000e+00; 0.000000000000000000e+00; 0.000000000000000000e+00; 4.000000000000000000e+00; 4.000000000000000000e+00; 4.000000000000000000e+00; 4.000000000000000000e+00; 4.000000000000000000e+00; 4.000000000000000000e+00; 4.000000000000000000e+00; 4.000000000000000000e+00}  SimLibPath=''  ClassIndex=1  ClassCtorIndex=0  ClassTabVisible=off  FunctionTabVisible=on  DelayDrawLabels=off  GraphFileSelect=Header file (*.h)  GraphHeaderFile=./aie/m16_ssr8_dft_graph.h  GraphClassName=m16_ssr8_dft_graph  GraphName=m16_ssr8_dft_graph  GraphHeaderFiles={'./aie/dft_1xN_widget_graph.h'; './aie/m16_ssr8_dft_graph.h'}  GraphSourceFile=./model_composer_work/xmc_aie_lib/8d40d72d/mygraph.cpp  GraphSearchPaths={'./aie'}  GraphPreProcOptions={}  blockJsonConstraints=[]
      | s[12;12;9;9;19;14;21;23;21;23;24;21;15;17;12;24;26;26;26;27;28;9;21;23;23;23;24;25;14;19;19;29]@FunctionNameDeclFileNamePortNamesPortTypesPortSerializedTypesPortDirectionsPortWindowSizeEnablesPortWindowMarginEnablesPortBufferSizeEnablesPortBufferMarginEnablesPortSynchronicityEnablesPortSignalSizeEnablesPortBufferSizesPortBufferMarginsFunctionDeclFunctionTemplateSpecKindFunctionTemplateParamNamesFunctionTemplateParamKindsFunctionTemplateParamTypesFunctionTemplateParamValuesFunctionTemplateParamEnablesClassDeclClassTemplateSpecKindClassTemplateParamNamesClassTemplateParamKindsClassTemplateParamTypesClassTemplateParamValuesClassTemplateParamEnablesClassCtorDeclsClassCtorParamNamesClassCtorParamTypesClassCtorParamSerializedTypes[1 1]@C[32 1]@nt30@../../aie/m16_ssr8_dft_graph.hC[2 1]@t5@sig_it5@sig_oC[2 1]@t48@std::array< adf::port< adf::direction::in >, 8 >t49@std::array< adf::port< adf::direction::out >, 8 >C[2 1]@t64@{Tstd::array{2{t{Tadf::port{1{t{Sadf::direction::in}}}}}{t{}8}}}t65@{Tstd::array{2{t{Tadf::port{1{t{Sadf::direction::out}}}}}{t{}8}}}C[2 1]@t5@inputt5@inputC[2 1]@l0@l0@C[2 1]@l0@l0@C[2 1]@l0@l0@C[2 1]@l0@l0@C[2 1]@l1@l1@C[2 1]@l0@l0@C[2 1]@nnC[2 1]@nnt139@void m16_ssr8_dft_graph::
      | (std::array< adf::port< adf::direction::in >, 8 > sig_i, std::array< adf::port< adf::direction::out >, 8 > sig_o)ne[0 1]@e[0 1]@e[0 1]@e[0 1]@e[0 1]@t25@class m16_ssr8_dft_graph;t4@nonee[0 1]@e[0 1]@e[0 1]@e[0 1]@e[0 1]@e[0 1]@e[0 1]@e[0 1]@e[0 1]@
  m16_ssr8_filterbank_graph : aieBasic/AIE Graph  PortAttributesTable={ 'Input', 'sig_i[0]', 'stream', 'cint16', '', '', ''; 'Input', 'sig_i[1]', 'stream', 'cint16', '', '', ''; 'Input', 'sig_i[2]', 'stream', 'cint16', '', '', ''; 'Input', 'sig_i[3]', 'stream', 'cint16', '', '', ''; 'Input', 'sig_i[4]', 'stream', 'cint16', '', '', ''; 'Input', 'sig_i[5]', 'stream', 'cint16', '', '', ''; 'Input', 'sig_i[6]', 'stream', 'cint16', '', '', ''; 'Input', 'sig_i[7]', 'stream', 'cint16', '', '', ''; 'Output', 'sig_o[0]', 'stream', 'cint16', '', '', '4'; 'Output', 'sig_o[1]', 'stream', 'cint16', '', '', '4'; 'Output', 'sig_o[2]', 'stream', 'cint16', '', '', '4'; 'Output', 'sig_o[3]', 'stream', 'cint16', '', '', '4'; 'Output', 'sig_o[4]', 'stream', 'cint16', '', '', '4'; 'Output', 'sig_o[5]', 'stream', 'cint16', '', '', '4'; 'Output', 'sig_o[6]', 'stream', 'cint16', '', '', '4'; 'Output', 'sig_o[7]', 'stream', 'cint16', '', '', '4' }  PortAttributesEnablement={'off', 'on', 'off', 'off', 'off', 'off', 'off';'off', 'on', 'off', 'off', 'off', 'off', 'off';'off', 'on', 'off', 'off', 'off', 'off', 'off';'off', 'on', 'off', 'off', 'off', 'off', 'off';'off', 'on', 'off', 'off', 'off', 'off', 'off';'off', 'on', 'off', 'off', 'off', 'off', 'off';'off', 'on', 'off', 'off', 'off', 'off', 'off';'off', 'on', 'off', 'off', 'off', 'off', 'off';'off', 'on', 'off', 'off', 'off', 'off', 'on';'off', 'on', 'off', 'off', 'off', 'off', 'on';'off', 'on', 'off', 'off', 'off', 'off', 'on';'off', 'on', 'off', 'off', 'off', 'off', 'on';'off', 'on', 'off', 'off', 'off', 'off', 'on';'off', 'on', 'off', 'off', 'off', 'off', 'on';'off', 'on', 'off', 'off', 'off', 'off', 'on';'off', 'on', 'off', 'off', 'off', 'off', 'on'}  SampleTime=-1  ClassDeclTypeOptions=C[1 1]@t31@class m16_ssr8_filterbank_graph  ClassDecl=class m16_ssr8_filterbank_graph  ClassTemplateParams={}  ClassTemplateParamsEnables={}  ClassCtorDeclTypeOptions=C[1 1]@t7@<empty>  ClassCtorDecl=<empty>  ClassCtorParams={}  GraphAllAttrs=|  PortArgDecls={'in stream cint16 in1'; 'in stream cint16 in2'; 'in stream cint16 in3'; 'in stream cint16 in4'; 'in stream cint16 in5'; 'in stream cint16 in6'; 'in stream cint16 in7'; 'in stream cint16 in8'; 'out stream cint16 out1'; 'out stream cint16 out2'; 'out stream cint16 out3'; 'out stream cint16 out4'; 'out stream cint16 out5'; 'out stream cint16 out6'; 'out stream cint16 out7'; 'out stream cint16 out8'}  PortGraphPortNames={'sig_i[0]'; 'sig_i[1]'; 'sig_i[2]'; 'sig_i[3]'; 'sig_i[4]'; 'sig_i[5]'; 'sig_i[6]'; 'sig_i[7]'; 'sig_o[0]'; 'sig_o[1]'; 'sig_o[2]'; 'sig_o[3]'; 'sig_o[4]'; 'sig_o[5]'; 'sig_o[6]'; 'sig_o[7]'}  PortTypes={'stream'; 'stream'; 'stream'; 'stream'; 'stream'; 'stream'; 'stream'; 'stream'; 'stream'; 'stream'; 'stream'; 'stream'; 'stream'; 'stream'; 'stream'; 'stream'}  PortDataTypes={'cint16'; 'cint16'; 'cint16'; 'cint16'; 'cint16'; 'cint16'; 'cint16'; 'cint16'; 'cint16'; 'cint16'; 'cint16'; 'cint16'; 'cint16'; 'cint16'; 'cint16'; 'cint16'}  PortSizes={0.000000000000000000e+00; 0.000000000000000000e+00; 0.000000000000000000e+00; 0.000000000000000000e+00; 0.000000000000000000e+00; 0.000000000000000000e+00; 0.000000000000000000e+00; 0.000000000000000000e+00; 0.000000000000000000e+00; 0.000000000000000000e+00; 0.000000000000000000e+00; 0.000000000000000000e+00; 0.000000000000000000e+00; 0.000000000000000000e+00; 0.000000000000000000e+00; 0.000000000000000000e+00}  PortSynchronicities={'auto'; 'auto'; 'auto'; 'auto'; 'auto'; 'auto'; 'auto'; 'auto'; 'auto'; 'auto'; 'auto'; 'auto'; 'auto'; 'auto'; 'auto'; 'auto'}  PortSignalSizes={0.000000000000000000e+00; 0.000000000000000000e+00; 0.000000000000000000e+00; 0.000000000000000000e+00; 0.000000000000000000e+00; 0.000000000000000000e+00; 0.000000000000000000e+00; 0.000000000000000000e+00; 4.000000000000000000e+00; 4.000000000000000000e+00; 4.000000000000000000e+00; 4.000000000000000000e+00; 4.000000000000000000e+00; 4.000000000000000000e+00; 4.000000000000000000e+00; 4.000000000000000000e+00}  SimLibPath=''  ClassIndex=1  ClassCtorIndex=0  ClassTabVisible=off  FunctionTabVisible=on  DelayDrawLabels=off  GraphFileSelect=Header file (*.h)  GraphHeaderFile=./aie/m16_ssr8_filterbank_graph.h  GraphClassName=m16_ssr8_filterbank_graph  GraphName=m16_ssr8_filterbank_graph  GraphHeaderFiles={'./aie/polyphase_fir_graph.h'; './aie/m16_ssr8_filterbank_graph.h'}  GraphSourceFile=./model_composer_work/xmc_aie_lib/fadd8e47/mygraph.cpp  GraphSearchPaths={'./aie'}  GraphPreProcOptions={}  blockJsonConstraints=[]
      | s[12;12;9;9;19;14;21;23;21;23;24;21;15;17;12;24;26;26;26;27;28;9;21;23;23;23;24;25;14;19;19;29]@FunctionNameDeclFileNamePortNamesPortTypesPortSerializedTypesPortDirectionsPortWindowSizeEnablesPortWindowMarginEnablesPortBufferSizeEnablesPortBufferMarginEnablesPortSynchronicityEnablesPortSignalSizeEnablesPortBufferSizesPortBufferMarginsFunctionDeclFunctionTemplateSpecKindFunctionTemplateParamNamesFunctionTemplateParamKindsFunctionTemplateParamTypesFunctionTemplateParamValuesFunctionTemplateParamEnablesClassDeclClassTemplateSpecKindClassTemplateParamNamesClassTemplateParamKindsClassTemplateParamTypesClassTemplateParamValuesClassTemplateParamEnablesClassCtorDeclsClassCtorParamNamesClassCtorParamTypesClassCtorParamSerializedTypes[1 1]@C[32 1]@nt37@../../aie/m16_ssr8_filterbank_graph.hC[2 1]@t5@sig_it5@sig_oC[2 1]@t48@std::array< adf::port< adf::direction::in >, 8 >t49@std::array< adf::port< adf::direction::out >, 8 >C[2 1]@t64@{Tstd::array{2{t{Tadf::port{1{t{Sadf::direction::in}}}}}{t{}8}}}t65@{Tstd::array{2{t{Tadf::port{1{t{Sadf::direction::out}}}}}{t{}8}}}C[2 1]@t5@inputt5@inputC[2 1]@l0@l0@C[2 1]@l0@l0@C[2 1]@l0@l0@C[2 1]@l0@l0@C[2 1]@l1@l1@C[2 1]@l0@l0@C[2 1]@nnC[2 1]@nnt146@void m16_ssr8_filterbank_graph::
      | (std::array< adf::port< adf::direction::in >, 8 > sig_i, std::array< adf::port< adf::direction::out >, 8 > sig_o)ne[0 1]@e[0 1]@e[0 1]@e[0 1]@e[0 1]@t32@class m16_ssr8_filterbank_graph;t4@nonee[0 1]@e[0 1]@e[0 1]@e[0 1]@e[0 1]@e[0 1]@e[0 1]@e[0 1]@e[0 1]@
  ChannelizerOut_0 : Outport
  ChannelizerOut_1 : Outport  Port=2
  ChannelizerOut_2 : Outport  Port=3
  ChannelizerOut_3 : Outport  Port=4
  ChannelizerOut_4 : Outport  Port=5
  ChannelizerOut_5 : Outport  Port=6
  ChannelizerOut_6 : Outport  Port=7
  ChannelizerOut_7 : Outport  Port=8
  ToOutputPermute_0 : Outport  Port=9
  ToOutputPermute_1 : Outport  Port=10
  ToOutputPermute_2 : Outport  Port=11
  ToOutputPermute_3 : Outport  Port=12
  ToOutputPermute_4 : Outport  Port=13
  ToOutputPermute_5 : Outport  Port=14
  ToOutputPermute_6 : Outport  Port=15
  ToOutputPermute_7 : Outport  Port=16
  wires:
  PLIO4/1 -> ToOutputPermute_3/1
  PLIO1/1 -> ToOutputPermute_0/1
  PLIO2/1 -> ToOutputPermute_1/1
  PLIO8/1 -> ToOutputPermute_7/1
  PLIO7/1 -> ToOutputPermute_6/1
  PLIO5/1 -> ToOutputPermute_4/1
  PLIO6/1 -> ToOutputPermute_5/1
  PLIO3/1 -> ToOutputPermute_2/1
  PLIO22/1 -> ChannelizerOut_6/1
  PLIO21/1 -> ChannelizerOut_5/1
  PLIO24/1 -> ChannelizerOut_0/1
  PLIO17/1 -> ChannelizerOut_1/1
  PLIO18/1 -> ChannelizerOut_2/1
  PLIO19/1 -> ChannelizerOut_3/1
  PLIO20/1 -> ChannelizerOut_4/1
  PLIO23/1 -> ChannelizerOut_7/1
  m16_ssr8_filterbank_graph/1 -> PLIO1/1
  m16_ssr8_filterbank_graph/7 -> PLIO7/1
  m16_ssr8_filterbank_graph/6 -> PLIO6/1
  PLIO59/1 -> m16_ssr8_filterbank_graph/4
  PLIO63/1 -> m16_ssr8_filterbank_graph/8
  FromInputPermute_0/1 -> PLIO48/1
  FromInputPermute_4/1 -> PLIO60/1
  PLIO61/1 -> m16_ssr8_filterbank_graph/6
  FromInputPermute_2/1 -> PLIO52/1
  PLIO52/1 -> m16_ssr8_filterbank_graph/3
  FromInputPermute_6/1 -> PLIO62/1
  FromInputPermute_5/1 -> PLIO61/1
  PLIO62/1 -> m16_ssr8_filterbank_graph/7
  FromInputPermute_3/1 -> PLIO59/1
  m16_ssr8_filterbank_graph/5 -> PLIO5/1
  FromInputPermute_7/1 -> PLIO63/1
  PLIO49/1 -> m16_ssr8_filterbank_graph/2
  m16_ssr8_filterbank_graph/8 -> PLIO8/1
  FromInputPermute_1/1 -> PLIO49/1
  PLIO60/1 -> m16_ssr8_filterbank_graph/5
  m16_ssr8_filterbank_graph/3 -> PLIO3/1
  PLIO48/1 -> m16_ssr8_filterbank_graph/1
  m16_ssr8_filterbank_graph/2 -> PLIO2/1
  m16_ssr8_filterbank_graph/4 -> PLIO4/1
  FromCyclicShift_3/1 -> PLIO14/1
  PLIO13/1 -> m16_ssr8_dft_graph/5
  m16_ssr8_dft_graph/8 -> PLIO23/1
  PLIO16/1 -> m16_ssr8_dft_graph/8
  FromCyclicShift_5/1 -> PLIO16/1
  m16_ssr8_dft_graph/1 -> PLIO24/1
  FromCyclicShift_2/1 -> PLIO13/1
  m16_ssr8_dft_graph/3 -> PLIO18/1
  FromCyclicShift_1/1 -> PLIO10/1
  m16_ssr8_dft_graph/6 -> PLIO21/1
  m16_ssr8_dft_graph/5 -> PLIO20/1
  PLIO12/1 -> m16_ssr8_dft_graph/4
  FromCyclicShift_7/1 -> PLIO12/1
  FromCyclicShift_6/1 -> PLIO11/1
  m16_ssr8_dft_graph/2 -> PLIO17/1
  FromCyclicShift_0/1 -> PLIO9/1
  PLIO10/1 -> m16_ssr8_dft_graph/2
  PLIO11/1 -> m16_ssr8_dft_graph/3
  PLIO9/1 -> m16_ssr8_dft_graph/1
  PLIO15/1 -> m16_ssr8_dft_graph/7
  FromCyclicShift_4/1 -> PLIO15/1
  m16_ssr8_dft_graph/4 -> PLIO19/1
  PLIO14/1 -> m16_ssr8_dft_graph/6
  m16_ssr8_dft_graph/7 -> PLIO22/1
